simulink model "PI_Level_Control"  (R2024b)
settings: Solver=VariableStepAuto  StartTime=0.0  StopTime=1000  RelTol=1e-3
values from neighbouring files (symbols this model uses):
  C = 6.8    [Arduino_Control_Script.m]    (also in PI_Level_Control_Script.m)
  k = 0.032    [Arduino_Control_Script.m]    (also in PI_Level_Control_Script.m)
  k1 = 0.624    [Arduino_Control_Script.m]    (also in PI_Level_Control_Script.m)
  k11 = k2^2+4*(k-k3)*k1    (= 0.0815946)    [Arduino_Control_Script.m]    (also in PI_Level_Control_Script.m)
  k12 = 8*(k-k3)    (= 0.2608)    [Arduino_Control_Script.m]    (also in PI_Level_Control_Script.m)
  k13 = 2*(k-k3)    (= 0.0652)    [Arduino_Control_Script.m]    (also in PI_Level_Control_Script.m)
  k2 = -0.015    [Arduino_Control_Script.m]    (also in PI_Level_Control_Script.m)
  k3 = -0.0006    [Arduino_Control_Script.m]    (also in PI_Level_Control_Script.m)
  keta = 8*10^-5    (= 8e-05)    [Arduino_Control_Script.m]    (also in PI_Level_Control_Script.m)
libraries: slpidlib x20
(part 3 of 3)

== system PI_Level_Control/Model Proces3/Motor ==
  um : Inport
  im : Inport  Port=2
  Add : Sum  Inputs=+-
  Rm : Gain  Gain=3
  kn : Outport
  wires:
  Rm/1 -> Add/2
  um/1 -> Add/1
  im/1 -> Rm/1
  Add/1 -> kn/1

== system PI_Level_Control/Model Proces3/Pompa ==
  kn : Inport
  h : Inport  Port=2
  Gain : Gain  Gain=k2
  Gain1 : Gain  Gain=k11
  Gain2 : Gain  Gain=k12
  Gain3 : Gain  Gain=1/k13
  Product : Product
  Sqrt : Sqrt
  Subtract : Sum  Inputs=+-
  Subtract1 : Sum
  q : Outport
  wires:
  Gain1/1 -> Subtract/1
  Gain2/1 -> Subtract/2
  Product/1 -> Gain1/1
  Gain/1 -> Subtract1/1
  kn/1 -> Product/2, Product/1, Gain/1
  Subtract/1 -> Sqrt/1
  Subtract1/1 -> Gain3/1
  Sqrt/1 -> Subtract1/2
  Gain3/1 -> q/1
  h/1 -> Gain2/1

== system PI_Level_Control/Model Proces3/Randament Pompa ==
  q : Inport
  um : Inport  Port=2
  Gain : Gain  Gain=keta
  Product : Product
  eta : Outport
  wires:
  Gain/1 -> Product/2
  Product/1 -> eta/1
  q/1 -> Product/1
  um/1 -> Gain/1

== system PI_Level_Control/Model Proces3/Rezervor ==
  q : Inport
  Add : Sum
  Constant : Constant  Value=C
  Gain : Gain  Gain=1/332.5
  Integrator : Integrator  InitialCondition=10.51
  Product : Product
  Product1 : Product
  Scope : Scope
  Sqrt : Sqrt
  Step : Step  Time=250  After=2  SampleTime=0
  Sum : Sum  Inputs=|+-
  h : Outport
  perturbatie : Outport  Port=2
  wires:
  Gain/1 -> Integrator/1
  Integrator/1 -> Sqrt/1, h/1
  Sum/1 -> Gain/1
  q/1 -> Sum/1
  Sqrt/1 -> Product1/1, Product/1
  Product/1 -> Scope/1, Sum/2
  Step/1 -> Product1/2, Add/1
  Constant/1 -> Add/2
  Add/1 -> Product/2
  Product1/1 -> perturbatie/1

== system PI_Level_Control/Model Proces4/Amplificator ==
  ua : Inport
  Constant : Constant  Value=8.1
  Gain : Gain  Gain=2.2
  Gain1 : Gain  Gain=2.2
  Gain2 : Gain  Gain=5
  Saturation : Saturate  UpperLimit=22  LowerLimit=0
  Sum : Sum  Inputs=|+-
  Sum1 : Sum  Inputs=|++
  Switch : Switch  Threshold=8.1  SaturateOnIntegerOverflow=off  InputSameDT=off
  um : Outport
  wires:
  ua/1 -> Gain/1, Sum/1, Gain1/1, Switch/2
  Gain1/1 -> Sum1/1
  Gain/1 -> Switch/3
  Sum1/1 -> Switch/1
  Gain2/1 -> Sum1/2
  Constant/1 -> Sum/2
  Switch/1 -> Saturation/1
  Sum/1 -> Gain2/1
  Saturation/1 -> um/1

== system PI_Level_Control/Model Proces4/Curent Rotoric ==
  h : Inport
  q : Inport  Port=2
  eta : Inport  Port=3
  um : Inport  Port=4
  Constant : Constant  Value=000.1
  Divide : Product  Inputs=**/
  Gain : Gain  Gain=2
  Gain1 : Gain  Gain=k
  Gain2 : Gain  Gain=1e+4
  Product : Product
  Product1 : Product
  Subtract : Sum
  Subtract1 : Sum
  im : Outport
  wires:
  Divide/1 -> im/1
  Subtract1/1 -> Divide/3
  Constant/1 -> Subtract1/1
  Gain2/1 -> Product1/1
  q/1 -> Divide/2, Product/1, Gain1/1
  Subtract/1 -> Divide/1
  Product/1 -> Subtract/2
  Gain/1 -> Subtract/1
  Gain1/1 -> Product/2
  Product1/1 -> Subtract1/2
  um/1 -> Product1/2
  h/1 -> Gain/1
  eta/1 -> Gain2/1

== system PI_Level_Control/Model Proces4/Filtru ==
  q : Inport
  Integrator : Integrator  InitialCondition=27.3
  Sum : Sum  Inputs=|+-
  q_f : Outport
  wires:
  Sum/1 -> Integrator/1
  Integrator/1 -> q_f/1, Sum/2
  q/1 -> Sum/1

== system PI_Level_Control/Model Proces4/Motor ==
  um : Inport
  im : Inport  Port=2
  Add : Sum  Inputs=+-
  Rm : Gain  Gain=3
  kn : Outport
  wires:
  Rm/1 -> Add/2
  um/1 -> Add/1
  im/1 -> Rm/1
  Add/1 -> kn/1

== system PI_Level_Control/Model Proces4/Pompa ==
  kn : Inport
  h : Inport  Port=2
  Gain : Gain  Gain=k2
  Gain1 : Gain  Gain=k11
  Gain2 : Gain  Gain=k12
  Gain3 : Gain  Gain=1/k13
  Product : Product
  Sqrt : Sqrt
  Subtract : Sum  Inputs=+-
  Subtract1 : Sum
  q : Outport
  wires:
  Gain1/1 -> Subtract/1
  Gain2/1 -> Subtract/2
  Product/1 -> Gain1/1
  Gain/1 -> Subtract1/1
  kn/1 -> Product/2, Product/1, Gain/1
  Subtract/1 -> Sqrt/1
  Subtract1/1 -> Gain3/1
  Sqrt/1 -> Subtract1/2
  Gain3/1 -> q/1
  h/1 -> Gain2/1

== system PI_Level_Control/Model Proces4/Randament Pompa ==
  q : Inport
  um : Inport  Port=2
  Gain : Gain  Gain=keta
  Product : Product
  eta : Outport
  wires:
  Gain/1 -> Product/2
  Product/1 -> eta/1
  q/1 -> Product/1
  um/1 -> Gain/1

== system PI_Level_Control/Model Proces4/Rezervor ==
  q : Inport
  Add : Sum
  Constant : Constant  Value=C
  Gain : Gain  Gain=1/332.5
  Integrator : Integrator  InitialCondition=16.02
  Product : Product
  Product1 : Product
  Scope : Scope
  Sqrt : Sqrt
  Step : Step  Time=250  After=2  SampleTime=0
  Sum : Sum  Inputs=|+-
  h : Outport
  perturbatie : Outport  Port=2
  wires:
  Gain/1 -> Integrator/1
  Integrator/1 -> Sqrt/1, h/1
  Sum/1 -> Gain/1
  q/1 -> Sum/1
  Sqrt/1 -> Product1/1, Product/1
  Product/1 -> Scope/1, Sum/2
  Step/1 -> Product1/2, Add/1
  Constant/1 -> Add/2
  Add/1 -> Product/2
  Product1/1 -> perturbatie/1

== system PI_Level_Control/Model Proces5/Amplificator ==
  ua : Inport
  Constant : Constant  Value=8.1
  Gain : Gain  Gain=2.2
  Gain1 : Gain  Gain=2.2
  Gain2 : Gain  Gain=5
  Saturation : Saturate  UpperLimit=22  LowerLimit=0
  Sum : Sum  Inputs=|+-
  Sum1 : Sum  Inputs=|++
  Switch : Switch  Threshold=8.1  SaturateOnIntegerOverflow=off  InputSameDT=off
  um : Outport
  wires:
  ua/1 -> Gain/1, Sum/1, Gain1/1, Switch/2
  Gain1/1 -> Sum1/1
  Gain/1 -> Switch/3
  Sum1/1 -> Switch/1
  Gain2/1 -> Sum1/2
  Constant/1 -> Sum/2
  Switch/1 -> Saturation/1
  Sum/1 -> Gain2/1
  Saturation/1 -> um/1

== system PI_Level_Control/Model Proces5/Curent Rotoric ==
  h : Inport
  q : Inport  Port=2
  eta : Inport  Port=3
  um : Inport  Port=4
  Constant : Constant  Value=000.1
  Divide : Product  Inputs=**/
  Gain : Gain  Gain=2
  Gain1 : Gain  Gain=k
  Gain2 : Gain  Gain=1e+4
  Product : Product
  Product1 : Product
  Subtract : Sum
  Subtract1 : Sum
  im : Outport
  wires:
  Divide/1 -> im/1
  Subtract1/1 -> Divide/3
  Constant/1 -> Subtract1/1
  Gain2/1 -> Product1/1
  q/1 -> Divide/2, Product/1, Gain1/1
  Subtract/1 -> Divide/1
  Product/1 -> Subtract/2
  Gain/1 -> Subtract/1
  Gain1/1 -> Product/2
  Product1/1 -> Subtract1/2
  um/1 -> Product1/2
  h/1 -> Gain/1
  eta/1 -> Gain2/1

== system PI_Level_Control/Model Proces5/Filtru ==
  q : Inport
  Integrator : Integrator  InitialCondition=29.2
  Sum : Sum  Inputs=|+-
  q_f : Outport
  wires:
  Sum/1 -> Integrator/1
  Integrator/1 -> q_f/1, Sum/2
  q/1 -> Sum/1

== system PI_Level_Control/Model Proces5/Motor ==
  um : Inport
  im : Inport  Port=2
  Add : Sum  Inputs=+-
  Rm : Gain  Gain=3
  kn : Outport
  wires:
  Rm/1 -> Add/2
  um/1 -> Add/1
  im/1 -> Rm/1
  Add/1 -> kn/1

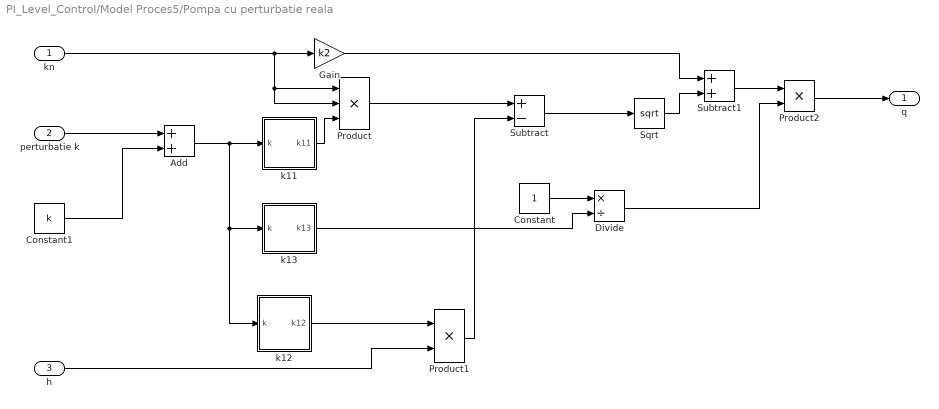
== system PI_Level_Control/Model Proces5/Pompa cu perturbatie reala ==
  kn : Inport
  perturbatie k : Inport  Port=2
  h : Inport  Port=3
  Add : Sum
  Constant : Constant
  Constant1 : Constant  Value=k
  Divide : Product  Inputs=*/
  Gain : Gain  Gain=k2
  Product : Product  Inputs=3
  Product1 : Product
  Product2 : Product
  Sqrt : Sqrt
  Subtract : Sum  Inputs=+-
  Subtract1 : Sum
  k11 : Subsystem
  k12 : Subsystem
  k13 : Subsystem
  q : Outport
  wires:
  h/1 -> Product1/2
  k12/1(k12) -> Product1/1
  Constant1/1 -> Add/2
  Add/1 -> k12/1(k), k13/1(k), k11/1(k)
  Gain/1 -> Subtract1/1
  Product/1 -> Subtract/1
  Divide/1 -> Product2/2
  kn/1 -> Product/2, Product/1, Gain/1
  Subtract/1 -> Sqrt/1
  k13/1(k13) -> Divide/2
  Subtract1/1 -> Product2/1
  k11/1(k11) -> Product/3
  Constant/1 -> Divide/1
  Product1/1 -> Subtract/2
  Sqrt/1 -> Subtract1/2
  perturbatie k/1 -> Add/1
  Product2/1 -> q/1

== system PI_Level_Control/Model Proces5/Randament Pompa ==
  q : Inport
  um : Inport  Port=2
  Gain : Gain  Gain=keta
  Product : Product
  eta : Outport
  wires:
  Gain/1 -> Product/2
  Product/1 -> eta/1
  q/1 -> Product/1
  um/1 -> Gain/1

== system PI_Level_Control/Model Proces5/Rezervor ==
  q : Inport
  Fcn : Fcn  Expr=sqrt(u)*9
  Gain : Gain  Gain=1/332.5
  Integrator : Integrator  InitialCondition=10.51
  Sum : Sum  Inputs=|+-
  h : Outport
  wires:
  Gain/1 -> Integrator/1
  Fcn/1 -> Sum/2
  Integrator/1 -> h/1, Fcn/1
  Sum/1 -> Gain/1
  q/1 -> Sum/1

== system PI_Level_Control/Model Proces6/Amplificator ==
  ua : Inport
  Constant : Constant  Value=8.1
  Gain : Gain  Gain=2.2
  Gain1 : Gain  Gain=2.2
  Gain2 : Gain  Gain=5
  Saturation : Saturate  UpperLimit=22  LowerLimit=0
  Sum : Sum  Inputs=|+-
  Sum1 : Sum  Inputs=|++
  Switch : Switch  Threshold=8.1  SaturateOnIntegerOverflow=off  InputSameDT=off
  um : Outport
  wires:
  ua/1 -> Gain/1, Sum/1, Gain1/1, Switch/2
  Gain1/1 -> Sum1/1
  Gain/1 -> Switch/3
  Sum1/1 -> Switch/1
  Gain2/1 -> Sum1/2
  Constant/1 -> Sum/2
  Switch/1 -> Saturation/1
  Sum/1 -> Gain2/1
  Saturation/1 -> um/1

== system PI_Level_Control/Model Proces6/Curent Rotoric ==
  h : Inport
  q : Inport  Port=2
  eta : Inport  Port=3
  um : Inport  Port=4
  Constant : Constant  Value=000.1
  Divide : Product  Inputs=**/
  Gain : Gain  Gain=2
  Gain1 : Gain  Gain=k
  Gain2 : Gain  Gain=1e+4
  Product : Product
  Product1 : Product
  Subtract : Sum
  Subtract1 : Sum
  im : Outport
  wires:
  Divide/1 -> im/1
  Subtract1/1 -> Divide/3
  Constant/1 -> Subtract1/1
  Gain2/1 -> Product1/1
  q/1 -> Divide/2, Product/1, Gain1/1
  Subtract/1 -> Divide/1
  Product/1 -> Subtract/2
  Gain/1 -> Subtract/1
  Gain1/1 -> Product/2
  Product1/1 -> Subtract1/2
  um/1 -> Product1/2
  h/1 -> Gain/1
  eta/1 -> Gain2/1

== system PI_Level_Control/Model Proces6/Filtru ==
  q : Inport
  Integrator : Integrator  InitialCondition=27.3
  Sum : Sum  Inputs=|+-
  q_f : Outport
  wires:
  Sum/1 -> Integrator/1
  Integrator/1 -> q_f/1, Sum/2
  q/1 -> Sum/1

== system PI_Level_Control/Model Proces6/Motor ==
  um : Inport
  im : Inport  Port=2
  Add : Sum  Inputs=+-
  Rm : Gain  Gain=3
  kn : Outport
  wires:
  Rm/1 -> Add/2
  um/1 -> Add/1
  im/1 -> Rm/1
  Add/1 -> kn/1

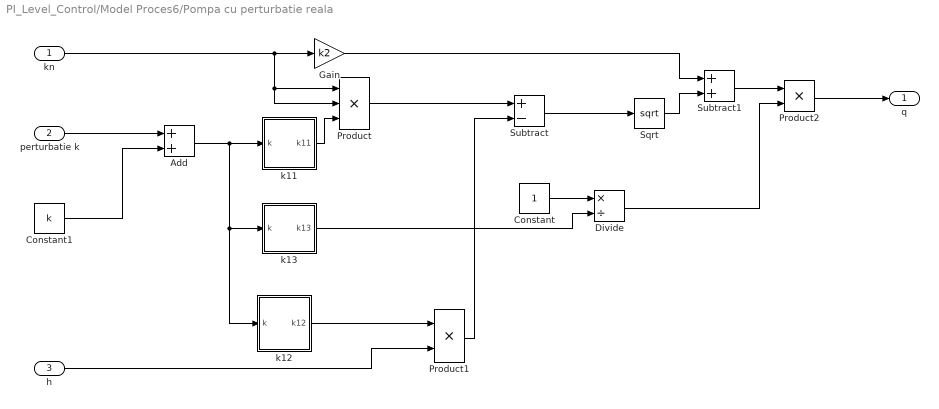
== system PI_Level_Control/Model Proces6/Pompa cu perturbatie reala ==
  kn : Inport
  perturbatie k : Inport  Port=2
  h : Inport  Port=3
  Add : Sum
  Constant : Constant
  Constant1 : Constant  Value=k
  Divide : Product  Inputs=*/
  Gain : Gain  Gain=k2
  Product : Product  Inputs=3
  Product1 : Product
  Product2 : Product
  Sqrt : Sqrt
  Subtract : Sum  Inputs=+-
  Subtract1 : Sum
  k11 : Subsystem
  k12 : Subsystem
  k13 : Subsystem
  q : Outport
  wires:
  h/1 -> Product1/2
  k12/1(k12) -> Product1/1
  Constant1/1 -> Add/2
  Add/1 -> k12/1(k), k13/1(k), k11/1(k)
  Gain/1 -> Subtract1/1
  Product/1 -> Subtract/1
  Divide/1 -> Product2/2
  kn/1 -> Product/2, Product/1, Gain/1
  Subtract/1 -> Sqrt/1
  k13/1(k13) -> Divide/2
  Subtract1/1 -> Product2/1
  k11/1(k11) -> Product/3
  Constant/1 -> Divide/1
  Product1/1 -> Subtract/2
  Sqrt/1 -> Subtract1/2
  perturbatie k/1 -> Add/1
  Product2/1 -> q/1

== system PI_Level_Control/Model Proces6/Randament Pompa ==
  q : Inport
  um : Inport  Port=2
  Gain : Gain  Gain=keta
  Product : Product
  eta : Outport
  wires:
  Gain/1 -> Product/2
  Product/1 -> eta/1
  q/1 -> Product/1
  um/1 -> Gain/1

== system PI_Level_Control/Model Proces6/Rezervor1 ==
  q : Inport
  Fcn : Fcn  Expr=sqrt(u)*6.8
  Gain : Gain  Gain=1/332.5
  Integrator : Integrator  InitialCondition=16.02
  Sum : Sum  Inputs=|+-
  h : Outport
  wires:
  Gain/1 -> Integrator/1
  Fcn/1 -> Sum/2
  Integrator/1 -> h/1, Fcn/1
  Sum/1 -> Gain/1
  q/1 -> Sum/1

== system PI_Level_Control/Model Proces7/Amplificator ==
  ua : Inport
  Constant : Constant  Value=8.1
  Gain : Gain  Gain=2.2
  Gain1 : Gain  Gain=2.2
  Gain2 : Gain  Gain=5
  Saturation : Saturate  UpperLimit=22  LowerLimit=0
  Sum : Sum  Inputs=|+-
  Sum1 : Sum  Inputs=|++
  Switch : Switch  Threshold=8.1  SaturateOnIntegerOverflow=off  InputSameDT=off
  um : Outport
  wires:
  ua/1 -> Gain/1, Sum/1, Gain1/1, Switch/2
  Gain1/1 -> Sum1/1
  Gain/1 -> Switch/3
  Sum1/1 -> Switch/1
  Gain2/1 -> Sum1/2
  Constant/1 -> Sum/2
  Switch/1 -> Saturation/1
  Sum/1 -> Gain2/1
  Saturation/1 -> um/1

== system PI_Level_Control/Model Proces7/Curent Rotoric ==
  h : Inport
  q : Inport  Port=2
  eta : Inport  Port=3
  um : Inport  Port=4
  Constant : Constant  Value=000.1
  Divide : Product  Inputs=**/
  Gain : Gain  Gain=2
  Gain1 : Gain  Gain=k
  Gain2 : Gain  Gain=1e+4
  Product : Product
  Product1 : Product
  Subtract : Sum
  Subtract1 : Sum
  im : Outport
  wires:
  Divide/1 -> im/1
  Subtract1/1 -> Divide/3
  Constant/1 -> Subtract1/1
  Gain2/1 -> Product1/1
  q/1 -> Divide/2, Product/1, Gain1/1
  Subtract/1 -> Divide/1
  Product/1 -> Subtract/2
  Gain/1 -> Subtract/1
  Gain1/1 -> Product/2
  Product1/1 -> Subtract1/2
  um/1 -> Product1/2
  h/1 -> Gain/1
  eta/1 -> Gain2/1

== system PI_Level_Control/Model Proces7/Filtru ==
  q : Inport
  Integrator : Integrator  InitialCondition=29.18
  Sum : Sum  Inputs=|+-
  q_f : Outport
  wires:
  Sum/1 -> Integrator/1
  Integrator/1 -> q_f/1, Sum/2
  q/1 -> Sum/1

== system PI_Level_Control/Model Proces7/Motor ==
  um : Inport
  im : Inport  Port=2
  Add : Sum  Inputs=+-
  Rm : Gain  Gain=3
  kn : Outport
  wires:
  Rm/1 -> Add/2
  um/1 -> Add/1
  im/1 -> Rm/1
  Add/1 -> kn/1

== system PI_Level_Control/Model Proces7/Pompa ==
  kn : Inport
  h : Inport  Port=2
  Gain : Gain  Gain=k2
  Gain1 : Gain  Gain=k11
  Gain2 : Gain  Gain=k12
  Gain3 : Gain  Gain=1/k13
  Product : Product
  Sqrt : Sqrt
  Subtract : Sum  Inputs=+-
  Subtract1 : Sum
  q : Outport
  wires:
  Gain1/1 -> Subtract/1
  Gain2/1 -> Subtract/2
  Product/1 -> Gain1/1
  Gain/1 -> Subtract1/1
  kn/1 -> Product/2, Product/1, Gain/1
  Subtract/1 -> Sqrt/1
  Subtract1/1 -> Gain3/1
  Sqrt/1 -> Subtract1/2
  Gain3/1 -> q/1
  h/1 -> Gain2/1

== system PI_Level_Control/Model Proces7/Randament Pompa ==
  q : Inport
  um : Inport  Port=2
  Gain : Gain  Gain=keta
  Product : Product
  eta : Outport
  wires:
  Gain/1 -> Product/2
  Product/1 -> eta/1
  q/1 -> Product/1
  um/1 -> Gain/1

== system PI_Level_Control/Model Proces7/Rezervor ==
  q : Inport
  Add : Sum
  Constant : Constant  Value=C
  Gain : Gain  Gain=1/332.5
  Integrator : Integrator  InitialCondition=10.51
  Product : Product
  Product1 : Product
  Scope : Scope
  Sqrt : Sqrt
  Step : Step  Time=500  After=2  SampleTime=0
  Sum : Sum  Inputs=|+-
  h : Outport
  perturbatie : Outport  Port=2
  wires:
  Gain/1 -> Integrator/1
  Integrator/1 -> Sqrt/1, h/1
  Sum/1 -> Gain/1
  q/1 -> Sum/1
  Sqrt/1 -> Product1/1, Product/1
  Product/1 -> Scope/1, Sum/2
  Step/1 -> Product1/2, Add/1
  Constant/1 -> Add/2
  Add/1 -> Product/2
  Product1/1 -> perturbatie/1

== system PI_Level_Control/Model Proces8/Amplificator ==
  ua : Inport
  Constant : Constant  Value=8.1
  Gain : Gain  Gain=2.2
  Gain1 : Gain  Gain=2.2
  Gain2 : Gain  Gain=5
  Saturation : Saturate  UpperLimit=22  LowerLimit=0
  Sum : Sum  Inputs=|+-
  Sum1 : Sum  Inputs=|++
  Switch : Switch  Threshold=8.1  SaturateOnIntegerOverflow=off  InputSameDT=off
  um : Outport
  wires:
  ua/1 -> Gain/1, Sum/1, Gain1/1, Switch/2
  Gain1/1 -> Sum1/1
  Gain/1 -> Switch/3
  Sum1/1 -> Switch/1
  Gain2/1 -> Sum1/2
  Constant/1 -> Sum/2
  Switch/1 -> Saturation/1
  Sum/1 -> Gain2/1
  Saturation/1 -> um/1

== system PI_Level_Control/Model Proces8/Curent Rotoric ==
  h : Inport
  q : Inport  Port=2
  eta : Inport  Port=3
  um : Inport  Port=4
  Constant : Constant  Value=000.1
  Divide : Product  Inputs=**/
  Gain : Gain  Gain=2
  Gain1 : Gain  Gain=k
  Gain2 : Gain  Gain=1e+4
  Product : Product
  Product1 : Product
  Subtract : Sum
  Subtract1 : Sum
  im : Outport
  wires:
  Divide/1 -> im/1
  Subtract1/1 -> Divide/3
  Constant/1 -> Subtract1/1
  Gain2/1 -> Product1/1
  q/1 -> Divide/2, Product/1, Gain1/1
  Subtract/1 -> Divide/1
  Product/1 -> Subtract/2
  Gain/1 -> Subtract/1
  Gain1/1 -> Product/2
  Product1/1 -> Subtract1/2
  um/1 -> Product1/2
  h/1 -> Gain/1
  eta/1 -> Gain2/1

== system PI_Level_Control/Model Proces8/Filtru ==
  q : Inport
  Integrator : Integrator  InitialCondition=27.3
  Sum : Sum  Inputs=|+-
  q_f : Outport
  wires:
  Sum/1 -> Integrator/1
  Integrator/1 -> q_f/1, Sum/2
  q/1 -> Sum/1

== system PI_Level_Control/Model Proces8/Motor ==
  um : Inport
  im : Inport  Port=2
  Add : Sum  Inputs=+-
  Rm : Gain  Gain=3
  kn : Outport
  wires:
  Rm/1 -> Add/2
  um/1 -> Add/1
  im/1 -> Rm/1
  Add/1 -> kn/1

== system PI_Level_Control/Model Proces8/Pompa ==
  kn : Inport
  h : Inport  Port=2
  Gain : Gain  Gain=k2
  Gain1 : Gain  Gain=k11
  Gain2 : Gain  Gain=k12
  Gain3 : Gain  Gain=1/k13
  Product : Product
  Sqrt : Sqrt
  Subtract : Sum  Inputs=+-
  Subtract1 : Sum
  q : Outport
  wires:
  Gain1/1 -> Subtract/1
  Gain2/1 -> Subtract/2
  Product/1 -> Gain1/1
  Gain/1 -> Subtract1/1
  kn/1 -> Product/2, Product/1, Gain/1
  Subtract/1 -> Sqrt/1
  Subtract1/1 -> Gain3/1
  Sqrt/1 -> Subtract1/2
  Gain3/1 -> q/1
  h/1 -> Gain2/1

== system PI_Level_Control/Model Proces8/Randament Pompa ==
  q : Inport
  um : Inport  Port=2
  Gain : Gain  Gain=keta
  Product : Product
  eta : Outport
  wires:
  Gain/1 -> Product/2
  Product/1 -> eta/1
  q/1 -> Product/1
  um/1 -> Gain/1

== system PI_Level_Control/Model Proces8/Rezervor ==
  q : Inport
  Add : Sum
  Constant : Constant  Value=C
  Gain : Gain  Gain=1/332.5
  Integrator : Integrator  InitialCondition=16.02
  Product : Product
  Product1 : Product
  Scope : Scope
  Sqrt : Sqrt
  Step : Step  Time=500  After=2  SampleTime=0
  Sum : Sum  Inputs=|+-
  h : Outport
  perturbatie : Outport  Port=2
  wires:
  Gain/1 -> Integrator/1
  Integrator/1 -> Sqrt/1, h/1
  Sum/1 -> Gain/1
  q/1 -> Sum/1
  Sqrt/1 -> Product1/1, Product/1
  Product/1 -> Scope/1, Sum/2
  Step/1 -> Product1/2, Add/1
  Constant/1 -> Add/2
  Add/1 -> Product/2
  Product1/1 -> perturbatie/1

== system PI_Level_Control/Model Proces9/Amplificator ==
  ua : Inport
  Constant : Constant  Value=8.1
  Gain : Gain  Gain=2.2
  Gain1 : Gain  Gain=2.2
  Gain2 : Gain  Gain=5
  Saturation : Saturate  UpperLimit=22  LowerLimit=0
  Sum : Sum  Inputs=|+-
  Sum1 : Sum  Inputs=|++
  Switch : Switch  Threshold=8.1  SaturateOnIntegerOverflow=off  InputSameDT=off
  um : Outport
  wires:
  ua/1 -> Gain/1, Sum/1, Gain1/1, Switch/2
  Gain1/1 -> Sum1/1
  Gain/1 -> Switch/3
  Sum1/1 -> Switch/1
  Gain2/1 -> Sum1/2
  Constant/1 -> Sum/2
  Switch/1 -> Saturation/1
  Sum/1 -> Gain2/1
  Saturation/1 -> um/1

== system PI_Level_Control/Model Proces9/Curent Rotoric ==
  h : Inport
  q : Inport  Port=2
  eta : Inport  Port=3
  um : Inport  Port=4
  Constant : Constant  Value=000.1
  Divide : Product  Inputs=**/
  Gain : Gain  Gain=2
  Gain1 : Gain  Gain=k
  Gain2 : Gain  Gain=1e+4
  Product : Product
  Product1 : Product
  Subtract : Sum
  Subtract1 : Sum
  im : Outport
  wires:
  Divide/1 -> im/1
  Subtract1/1 -> Divide/3
  Constant/1 -> Subtract1/1
  Gain2/1 -> Product1/1
  q/1 -> Divide/2, Product/1, Gain1/1
  Subtract/1 -> Divide/1
  Product/1 -> Subtract/2
  Gain/1 -> Subtract/1
  Gain1/1 -> Product/2
  Product1/1 -> Subtract1/2
  um/1 -> Product1/2
  h/1 -> Gain/1
  eta/1 -> Gain2/1

== system PI_Level_Control/Model Proces9/Filtru ==
  q : Inport
  Integrator : Integrator  InitialCondition=29.18
  Sum : Sum  Inputs=|+-
  q_f : Outport
  wires:
  Sum/1 -> Integrator/1
  Integrator/1 -> q_f/1, Sum/2
  q/1 -> Sum/1

== system PI_Level_Control/Model Proces9/Motor ==
  um : Inport
  im : Inport  Port=2
  Add : Sum  Inputs=+-
  Rm : Gain  Gain=3
  kn : Outport
  wires:
  Rm/1 -> Add/2
  um/1 -> Add/1
  im/1 -> Rm/1
  Add/1 -> kn/1

== system PI_Level_Control/Model Proces9/Pompa ==
  kn : Inport
  h : Inport  Port=2
  Gain : Gain  Gain=k2
  Gain1 : Gain  Gain=k11
  Gain2 : Gain  Gain=k12
  Gain3 : Gain  Gain=1/k13
  Product : Product
  Sqrt : Sqrt
  Subtract : Sum  Inputs=+-
  Subtract1 : Sum
  q : Outport
  wires:
  Gain1/1 -> Subtract/1
  Gain2/1 -> Subtract/2
  Product/1 -> Gain1/1
  Gain/1 -> Subtract1/1
  kn/1 -> Product/2, Product/1, Gain/1
  Subtract/1 -> Sqrt/1
  Subtract1/1 -> Gain3/1
  Sqrt/1 -> Subtract1/2
  Gain3/1 -> q/1
  h/1 -> Gain2/1

== system PI_Level_Control/Model Proces9/Randament Pompa ==
  q : Inport
  um : Inport  Port=2
  Gain : Gain  Gain=keta
  Product : Product
  eta : Outport
  wires:
  Gain/1 -> Product/2
  Product/1 -> eta/1
  q/1 -> Product/1
  um/1 -> Gain/1

== system PI_Level_Control/Model Proces9/Rezervor ==
  q : Inport
  Fcn : Fcn  Expr=sqrt(u)*9
  Gain : Gain  Gain=1/332.5
  Integrator : Integrator  InitialCondition=10.51
  Sum : Sum  Inputs=|+-
  h : Outport
  wires:
  Gain/1 -> Integrator/1
  Fcn/1 -> Sum/2
  Integrator/1 -> h/1, Fcn/1
  Sum/1 -> Gain/1
  q/1 -> Sum/1

== system PI_Level_Control/Model Proces10/Pompa cu perturbatie reala/k11 ==
  k : Inport
  Add : Sum
  Constant : Constant  Value=k2
  Constant1 : Constant  Value=k1
  Constant2 : Constant  Value=k3
  Constant3 : Constant  Value=4
  Display : Display
  Power : Math  Operator=square
  Product : Product  Inputs=3
  Subtract : Sum  Inputs=+-
  k11 : Outport
  wires:
  Constant/1 -> Power/1
  Power/1 -> Display/1, Add/1
  k/1 -> Subtract/1
  Constant2/1 -> Subtract/2
  Subtract/1 -> Product/1
  Constant1/1 -> Product/2
  Constant3/1 -> Product/3
  Product/1 -> Add/2
  Add/1 -> k11/1

== system PI_Level_Control/Model Proces10/Pompa cu perturbatie reala/k12 ==
  k : Inport
  Constant : Constant  Value=8
  Constant1 : Constant  Value=k3
  Display1 : Display
  Product : Product
  Subtract : Sum  Inputs=+-
  k12 : Outport
  wires:
  k/1 -> Subtract/1
  Subtract/1 -> Product/1
  Constant1/1 -> Subtract/2
  Constant/1 -> Product/2
  Product/1 -> k12/1, Display1/1

== system PI_Level_Control/Model Proces10/Pompa cu perturbatie reala/k13 ==
  k : Inport
  Constant : Constant  Value=2
  Constant1 : Constant  Value=k3
  Display : Display
  Product : Product
  Subtract : Sum  Inputs=+-
  k13 : Outport
  wires:
  k/1 -> Subtract/1
  Constant/1 -> Product/1
  Constant1/1 -> Subtract/2
  Subtract/1 -> Product/2
  Product/1 -> k13/1, Display/1

== system PI_Level_Control/Model Proces11/Pompa cu perturbatie reala/k11 ==
  k : Inport
  Add : Sum
  Constant : Constant  Value=k2
  Constant1 : Constant  Value=k1
  Constant2 : Constant  Value=k3
  Constant3 : Constant  Value=4
  Display : Display
  Power : Math  Operator=square
  Product : Product  Inputs=3
  Subtract : Sum  Inputs=+-
  k11 : Outport
  wires:
  Constant/1 -> Power/1
  Power/1 -> Display/1, Add/1
  k/1 -> Subtract/1
  Constant2/1 -> Subtract/2
  Subtract/1 -> Product/1
  Constant1/1 -> Product/2
  Constant3/1 -> Product/3
  Product/1 -> Add/2
  Add/1 -> k11/1

== system PI_Level_Control/Model Proces11/Pompa cu perturbatie reala/k12 ==
  k : Inport
  Constant : Constant  Value=8
  Constant1 : Constant  Value=k3
  Display1 : Display
  Product : Product
  Subtract : Sum  Inputs=+-
  k12 : Outport
  wires:
  k/1 -> Subtract/1
  Subtract/1 -> Product/1
  Constant1/1 -> Subtract/2
  Constant/1 -> Product/2
  Product/1 -> k12/1, Display1/1

== system PI_Level_Control/Model Proces11/Pompa cu perturbatie reala/k13 ==
  k : Inport
  Constant : Constant  Value=2
  Constant1 : Constant  Value=k3
  Display : Display
  Product : Product
  Subtract : Sum  Inputs=+-
  k13 : Outport
  wires:
  k/1 -> Subtract/1
  Constant/1 -> Product/1
  Constant1/1 -> Subtract/2
  Subtract/1 -> Product/2
  Product/1 -> k13/1, Display/1

== system PI_Level_Control/Model Proces12/Pompa cu perturbatie reala/k11 ==
  k : Inport
  Add : Sum
  Constant : Constant  Value=k2
  Constant1 : Constant  Value=k1
  Constant2 : Constant  Value=k3
  Constant3 : Constant  Value=4
  Display : Display
  Power : Math  Operator=square
  Product : Product  Inputs=3
  Subtract : Sum  Inputs=+-
  k11 : Outport
  wires:
  Constant/1 -> Power/1
  Power/1 -> Display/1, Add/1
  k/1 -> Subtract/1
  Constant2/1 -> Subtract/2
  Subtract/1 -> Product/1
  Constant1/1 -> Product/2
  Constant3/1 -> Product/3
  Product/1 -> Add/2
  Add/1 -> k11/1

== system PI_Level_Control/Model Proces12/Pompa cu perturbatie reala/k12 ==
  k : Inport
  Constant : Constant  Value=8
  Constant1 : Constant  Value=k3
  Display1 : Display
  Product : Product
  Subtract : Sum  Inputs=+-
  k12 : Outport
  wires:
  k/1 -> Subtract/1
  Subtract/1 -> Product/1
  Constant1/1 -> Subtract/2
  Constant/1 -> Product/2
  Product/1 -> k12/1, Display1/1

== system PI_Level_Control/Model Proces12/Pompa cu perturbatie reala/k13 ==
  k : Inport
  Constant : Constant  Value=2
  Constant1 : Constant  Value=k3
  Display : Display
  Product : Product
  Subtract : Sum  Inputs=+-
  k13 : Outport
  wires:
  k/1 -> Subtract/1
  Constant/1 -> Product/1
  Constant1/1 -> Subtract/2
  Subtract/1 -> Product/2
  Product/1 -> k13/1, Display/1

== system PI_Level_Control/Model Proces13/Pompa cu perturbatie reala/k11 ==
  k : Inport
  Add : Sum
  Constant : Constant  Value=k2
  Constant1 : Constant  Value=k1
  Constant2 : Constant  Value=k3
  Constant3 : Constant  Value=4
  Display : Display
  Power : Math  Operator=square
  Product : Product  Inputs=3
  Subtract : Sum  Inputs=+-
  k11 : Outport
  wires:
  Constant/1 -> Power/1
  Power/1 -> Display/1, Add/1
  k/1 -> Subtract/1
  Constant2/1 -> Subtract/2
  Subtract/1 -> Product/1
  Constant1/1 -> Product/2
  Constant3/1 -> Product/3
  Product/1 -> Add/2
  Add/1 -> k11/1

== system PI_Level_Control/Model Proces13/Pompa cu perturbatie reala/k12 ==
  k : Inport
  Constant : Constant  Value=8
  Constant1 : Constant  Value=k3
  Display1 : Display
  Product : Product
  Subtract : Sum  Inputs=+-
  k12 : Outport
  wires:
  k/1 -> Subtract/1
  Subtract/1 -> Product/1
  Constant1/1 -> Subtract/2
  Constant/1 -> Product/2
  Product/1 -> k12/1, Display1/1

== system PI_Level_Control/Model Proces13/Pompa cu perturbatie reala/k13 ==
  k : Inport
  Constant : Constant  Value=2
  Constant1 : Constant  Value=k3
  Display : Display
  Product : Product
  Subtract : Sum  Inputs=+-
  k13 : Outport
  wires:
  k/1 -> Subtract/1
  Constant/1 -> Product/1
  Constant1/1 -> Subtract/2
  Subtract/1 -> Product/2
  Product/1 -> k13/1, Display/1

== system PI_Level_Control/Model Proces5/Pompa cu perturbatie reala/k11 ==
  k : Inport
  Add : Sum
  Constant : Constant  Value=k2
  Constant1 : Constant  Value=k1
  Constant2 : Constant  Value=k3
  Constant3 : Constant  Value=4
  Display : Display
  Power : Math  Operator=square
  Product : Product  Inputs=3
  Subtract : Sum  Inputs=+-
  k11 : Outport
  wires:
  Constant/1 -> Power/1
  Power/1 -> Display/1, Add/1
  k/1 -> Subtract/1
  Constant2/1 -> Subtract/2
  Subtract/1 -> Product/1
  Constant1/1 -> Product/2
  Constant3/1 -> Product/3
  Product/1 -> Add/2
  Add/1 -> k11/1

== system PI_Level_Control/Model Proces5/Pompa cu perturbatie reala/k12 ==
  k : Inport
  Constant : Constant  Value=8
  Constant1 : Constant  Value=k3
  Display1 : Display
  Product : Product
  Subtract : Sum  Inputs=+-
  k12 : Outport
  wires:
  k/1 -> Subtract/1
  Subtract/1 -> Product/1
  Constant1/1 -> Subtract/2
  Constant/1 -> Product/2
  Product/1 -> k12/1, Display1/1

== system PI_Level_Control/Model Proces5/Pompa cu perturbatie reala/k13 ==
  k : Inport
  Constant : Constant  Value=2
  Constant1 : Constant  Value=k3
  Display : Display
  Product : Product
  Subtract : Sum  Inputs=+-
  k13 : Outport
  wires:
  k/1 -> Subtract/1
  Constant/1 -> Product/1
  Constant1/1 -> Subtract/2
  Subtract/1 -> Product/2
  Product/1 -> k13/1, Display/1

== system PI_Level_Control/Model Proces6/Pompa cu perturbatie reala/k11 ==
  k : Inport
  Add : Sum
  Constant : Constant  Value=k2
  Constant1 : Constant  Value=k1
  Constant2 : Constant  Value=k3
  Constant3 : Constant  Value=4
  Display : Display
  Power : Math  Operator=square
  Product : Product  Inputs=3
  Subtract : Sum  Inputs=+-
  k11 : Outport
  wires:
  Constant/1 -> Power/1
  Power/1 -> Display/1, Add/1
  k/1 -> Subtract/1
  Constant2/1 -> Subtract/2
  Subtract/1 -> Product/1
  Constant1/1 -> Product/2
  Constant3/1 -> Product/3
  Product/1 -> Add/2
  Add/1 -> k11/1

== system PI_Level_Control/Model Proces6/Pompa cu perturbatie reala/k12 ==
  k : Inport
  Constant : Constant  Value=8
  Constant1 : Constant  Value=k3
  Display1 : Display
  Product : Product
  Subtract : Sum  Inputs=+-
  k12 : Outport
  wires:
  k/1 -> Subtract/1
  Subtract/1 -> Product/1
  Constant1/1 -> Subtract/2
  Constant/1 -> Product/2
  Product/1 -> k12/1, Display1/1

== system PI_Level_Control/Model Proces6/Pompa cu perturbatie reala/k13 ==
  k : Inport
  Constant : Constant  Value=2
  Constant1 : Constant  Value=k3
  Display : Display
  Product : Product
  Subtract : Sum  Inputs=+-
  k13 : Outport
  wires:
  k/1 -> Subtract/1
  Constant/1 -> Product/1
  Constant1/1 -> Subtract/2
  Subtract/1 -> Product/2
  Product/1 -> k13/1, Display/1
